simulink model "Microgrid_transition_model_092221"  (R2020a)
settings: Solver=VariableStepAuto  StartTime=0.0  StopTime=16  MaxStep=1e-4  RelTol=1e-3
PreLoadFcn:
  | %run('FC_microgrid_param.m')
  | %load('gen_grid_init.mat')
InitFcn:
  | %load myisoModel_init;
  | run('FC_microgrid_param.m')
  | tic
  | run('CARTinitFcn.m')
  | %caseNo = 2;
  | 
  | %if (caseNo == 1)
  | %set_param(['Isolated_grid_paper_model_022521/SignalGen'], 'ActiveScenario', 'PStep222kW');
  | %else
  | %set_param(['Isolated_grid_paper_model_022521/SignalGen'], 'ActiveScenario', 'QStep222kVAr');
  | 
  | %end;
StopFcn:
  | toc
undefined symbols (not defined in the file): breakpoints1, breakpoints2, cp_table_data, ctrl, D1, Delta, DiscIntNeverNeededParam, DT, FC_BESS, find_system, gcbh, libFC_BESS, LowerLimit, magnitude, oversize, pq_ts, sps_rtmsupport, timer, ts, Ts, Ts_APC, Ts_Control, Ts_Power, UpperLimit
libraries: powerlib x120, powerlib_meascontrol x85, simulink x63, powerlib_extras x40, simulink_extras x12, eePowerMeasurement x9, sps_avr x7, pi_ctrl x4, spsDieselMotorModel x3, SignalEditorBlockLib x2, libLgBattery x1, libFC_PV x1
(part 8 of 11)

== system Microgrid_transition_model_092221/../Control/Grid-side converter Control system/INT ==
  note: INTEGRATOR (Trapezoidal) with External limits & Reset & Hold
  Max : Inport
  Min : Inport  Port=2
  In : Inport  Port=3
  Ki : Inport  Port=4
  Hold : Inport  Port=5
  Reset : Inport  Port=6
  Reset Value : Inport  Port=7
  Gain : Gain  Gain=Ts* 0.5  SaturateOnIntegerOverflow=on  OutDataTypeStr=Inherit: Same as input  ParamDataTypeStr=Inherit: Same as input
  IC = 0 : UnitDelay  SampleTime=Ts  HasFrameUpgradeWarning=on
  IC = i_ic : UnitDelay  SampleTime=Ts  HasFrameUpgradeWarning=on
  Logical Operator4 : Logic  Operator=OR
  MinMax : MinMax  Inputs=2  InputSameDT=on  SaturateOnIntegerOverflow=on
  MinMax1 : MinMax  Function=max  Inputs=2  InputSameDT=on  SaturateOnIntegerOverflow=on
  Product : Product  SaturateOnIntegerOverflow=on  OutDataTypeStr=Inherit: Same as first input
  S6 : Subsystem  mask(Limiter with External Limits){}
      mask Display: disp('      Limiter\n')
  Sum : Sum  InputSameDT=on  SaturateOnIntegerOverflow=on  OutDataTypeStr=Inherit: Same as first input
  Sum1 : Sum  InputSameDT=on  SaturateOnIntegerOverflow=on  OutDataTypeStr=Inherit: Same as first input
  Switch2 : Switch  Threshold=0.5  SaturateOnIntegerOverflow=on  InputSameDT=on
  Switch3 : Switch  Threshold=0.5  SaturateOnIntegerOverflow=on  InputSameDT=on
  Switch7 : Switch  Threshold=0.5  SaturateOnIntegerOverflow=on  InputSameDT=on
  Out : Outport  InitialOutput=0  VectorParamsAs1DForOutWhenUnconnected=off
  wires:
  S6/1("  ") -> IC = i_ic/1, Out/1
  Gain/1 -> Product/1
  Sum1/1 -> Product/2
  Ki/1 -> Gain/1
  IC = 0/1 -> Sum1/2
  In/1 -> IC = 0/1, Sum1/1
  Product/1 -> Sum/1
  Sum/1 -> S6/2(In)
  Hold/1 -> Logical Operator4/1
  Reset/1 -> Switch7/2, Logical Operator4/2
  Logical Operator4/1 -> Switch2/2, Switch3/2
  Switch2/1 -> MinMax/1
  Max/1 -> Switch2/3, MinMax/2
  Reset Value/1 -> Switch7/1
  MinMax/1 -> S6/1(MAX)
  MinMax1/1 -> S6/3(MIN)
  Switch3/1 -> MinMax1/1
  Min/1 -> Switch3/3, MinMax1/2
  IC = i_ic/1 -> Switch7/3
  Switch7/1 -> Switch2/1, Sum/2, Switch3/1

== system Microgrid_transition_model_092221/../Control/Measurement and Transformation/Discrete 3-phase PLL-Driven Positive-Sequence Active & Reactive Power ==
  note: Discrete 3-phase PLL-driven Positive-Sequence Active & Reactive Power
  note: Pierre Giroux, Gilbert Sybille
      | Power System Simulation Laboratory
      | IREQ, Hydro-Quebc
  Freq : Inport  PortDimensions=1
  w : Inport  Port=2  PortDimensions=1
  Vabc : Inport  Port=3  PortDimensions=3
  Iabc : Inport  Port=4  PortDimensions=3
  Deg->Rad : Gain  Gain=pi/180  SaturateOnIntegerOverflow=on  OutDataTypeStr=Inherit: Same as input  ParamDataTypeStr=Inherit: Same as input
  Discrete 3-phase PLL-Driven Positive-Sequence Fundamental Value : Subsystem  mask(Discrete 3-phase PLL-Driven Positive-Sequence Fundamental Value){Finit=Finit, Fmin=Fmin, Par_Init=Par_Vinit, Ts=Ts}
      mask prompts: Finit "Initial frequency (Hz):"; Fmin "Minimum frequency (Hz):"; Par_Init "Initial input (positive component): [ Mag  Phase-relative-to-PLL(degrees) ]"; Ts "Sample time:"
      mask help:
      | For a supplied fundamental frequency (port Freq), this discrete block computes  the positive-sequence component (Magnitude and Phase)  of a set of three balanced or unbalanced signals (port abc) which may contain harmonics.
      |  Input port "Sin_Cos" (a two-dimension signal) provides the reference frame required for the computation..
      |  First and second outputs return respectively the magnitude and phase (in degrees relative to the PLL phase)) of the fundamental.
      | For the first cycle of simulation, the outputs are held constant to the values specified by the parameter "Initial input".
      | constant to the values specified by the parameter "Initial input". The value of the parameter "Minimum frequency" is used to determine the buffer size of the "Variable Transport Delay" block found inside this subsystem.
      mask init:
      | Real_Init=Par_Init(1)*cos(pi/180*Par_Init(2));
      | Imag_Init=Par_Init(1)*sin(pi/180*Par_Init(2));
      | power_initmask();
      settings: OpenFcn=power_openblockproxy();
  Discrete 3-phase PLL-Driven Positive-Sequence Fundamental Value2 : Subsystem  mask(Discrete 3-phase PLL-Driven Positive-Sequence Fundamental Value){Finit=Finit, Fmin=Fmin, Par_Init=Par_Iinit, Ts=Ts}
      mask prompts: Finit "Initial frequency (Hz):"; Fmin "Minimum frequency (Hz):"; Par_Init "Initial input (positive component): [ Mag  Phase-relative-to-PLL(degrees) ]"; Ts "Sample time:"
      mask help:
      | For a supplied fundamental frequency (port Freq), this discrete block computes  the positive-sequence component (Magnitude and Phase)  of a set of three balanced or unbalanced signals (port abc) which may contain harmonics.
      |  Input port "Sin_Cos" (a two-dimension signal) provides the reference frame required for the computation..
      |  First and second outputs return respectively the magnitude and phase (in degrees relative to the PLL phase)) of the fundamental.
      | For the first cycle of simulation, the outputs are held constant to the values specified by the parameter "Initial input".
      | constant to the values specified by the parameter "Initial input". The value of the parameter "Minimum frequency" is used to determine the buffer size of the "Variable Transport Delay" block found inside this subsystem.
      mask init:
      | Real_Init=Par_Init(1)*cos(pi/180*Par_Init(2));
      | Imag_Init=Par_Init(1)*sin(pi/180*Par_Init(2));
      | power_initmask();
      settings: OpenFcn=power_openblockproxy();
  Gain1 : Gain  Gain=3/2  SaturateOnIntegerOverflow=on  OutDataTypeStr=Inherit: Same as input  ParamDataTypeStr=Inherit: Same as input
  Mux2 : Mux  Inputs=2
  Mux3 : Mux  Inputs=2
  Product : Product  InputSameDT=on  SaturateOnIntegerOverflow=on  OutDataTypeStr=Inherit: Same as first input
  Product1 : Product  InputSameDT=on  SaturateOnIntegerOverflow=on  OutDataTypeStr=Inherit: Same as first input
  Product2 : Product  InputSameDT=on  SaturateOnIntegerOverflow=on  OutDataTypeStr=Inherit: Same as first input
  Sum : Sum  Inputs=+-  InputSameDT=on  SaturateOnIntegerOverflow=on  OutDataTypeStr=Inherit: Same as first input
  Trigonometric Function : Trigonometry
  Trigonometric Function1 : Trigonometry  Operator=cos
  Mag_V_I : Outport  VectorParamsAs1DForOutWhenUnconnected=off
  P_Q : Outport  Port=2  VectorParamsAs1DForOutWhenUnconnected=off
  wires:
  Vabc/1 -> Discrete 3-phase PLL-Driven Positive-Sequence Fundamental Value/3(abc)
  Freq/1 -> Discrete 3-phase PLL-Driven Positive-Sequence Fundamental Value/1(Freq), Discrete 3-phase PLL-Driven Positive-Sequence Fundamental Value2/1(Freq)
  w/1 -> Discrete 3-phase PLL-Driven Positive-Sequence Fundamental Value/2(w), Discrete 3-phase PLL-Driven Positive-Sequence Fundamental Value2/2(w)
  Discrete 3-phase PLL-Driven Positive-Sequence Fundamental Value/2(Phase) -> Sum/1
  Discrete 3-phase PLL-Driven Positive-Sequence Fundamental Value/1(Mag) -> Mux3/1, Product2/1
  Discrete 3-phase PLL-Driven Positive-Sequence Fundamental Value2/2(Phase) -> Sum/2
  Sum/1 -> Deg->Rad/1
  Deg->Rad/1 -> Trigonometric Function1/1, Trigonometric Function/1
  Trigonometric Function1/1 -> Product/2
  Trigonometric Function/1 -> Product1/1
  Mux2/1 -> Gain1/1
  Product/1 -> Mux2/1
  Product1/1 -> Mux2/2
  Mux3/1 -> Mag_V_I/1
  Gain1/1 -> P_Q/1
  Product2/1 -> Product/1, Product1/2
  Discrete 3-phase PLL-Driven Positive-Sequence Fundamental Value2/1(Mag) -> Mux3/2, Product2/2
  Iabc/1 -> Discrete 3-phase PLL-Driven Positive-Sequence Fundamental Value2/3(abc)

== system Microgrid_transition_model_092221/../Control/Measurement and Transformation/Filter ==
  Vabc_grid : Inport
  Iabc_grid_conv : Inport  Port=2
  Vabc_LL_s : Inport  Port=3
  Iabc_stator : Inport  Port=4
  IL : Inport  Port=5
  Vdc : Inport  Port=6
  Qref : Inport  Port=7
  wr : Inport  Port=8
  angle_rotor : Inport  Port=9
  Second-Order Filter{,1..6} (7 alike) : powerlib_meascontrol/Filters/Second-Order Filter  FilterType=Lowpass  Fo=Freq  Zeta=Zeta  Ts=Ts  Initialize=off  Vac_Init="[0,  0,  60]"  Vdc_Init=0  PlotResponse=off  FreqRange=[0, 500, 1]
      settings: SourceProductBaseCode=MT,PS
  Second-Order Filter7 : powerlib_meascontrol/Filters/Second-Order Filter  FilterType=Lowpass  Fo=Freq  Zeta=Zeta  Ts=Ts  Initialize=on  Vac_Init=[0.8 -25 60]*0  Vdc_Init=Vdc_nom  PlotResponse=off  FreqRange=[0, 500, 1]
      settings: SourceProductBaseCode=MT,PS
  Second-Order Filter8 : powerlib_meascontrol/Filters/Second-Order Filter  FilterType=Lowpass  Fo=Freq  Zeta=Zeta  Ts=Ts  Initialize=on  Vac_Init=[0.8 -25 60]*0  Vdc_Init=1+init(1)/100  PlotResponse=off  FreqRange=[0, 500, 1]
      settings: SourceProductBaseCode=MT,PS
  "Vabc_grid " : Outport  VectorParamsAs1DForOutWhenUnconnected=off
  "Iabc_grid_conv " : Outport  Port=2  VectorParamsAs1DForOutWhenUnconnected=off
  "Vabc_LL_s " : Outport  Port=3  VectorParamsAs1DForOutWhenUnconnected=off
  "Iabc_stator " : Outport  Port=4  VectorParamsAs1DForOutWhenUnconnected=off
  "IL " : Outport  Port=5  VectorParamsAs1DForOutWhenUnconnected=off
  "Vdc " : Outport  Port=6  VectorParamsAs1DForOutWhenUnconnected=off
  "Qref " : Outport  Port=7  VectorParamsAs1DForOutWhenUnconnected=off
  "wr " : Outport  Port=8  VectorParamsAs1DForOutWhenUnconnected=off
  "angle_rotor " : Outport  Port=9  VectorParamsAs1DForOutWhenUnconnected=off
  wires:
  Iabc_stator/1 -> Second-Order Filter3/1
  Second-Order Filter2/1 -> "Vabc_LL_s "/1
  Vabc_LL_s/1 -> Second-Order Filter2/1
  Iabc_grid_conv/1 -> Second-Order Filter1/1
  Vabc_grid/1 -> Second-Order Filter/1
  Second-Order Filter4/1 -> "IL "/1
  IL/1 -> Second-Order Filter4/1
  Second-Order Filter5/1 -> "Qref "/1
  Qref/1 -> Second-Order Filter5/1
  Second-Order Filter8/1 -> "wr "/1
  wr/1 -> Second-Order Filter8/1
  Second-Order Filter3/1 -> "Iabc_stator "/1
  Second-Order Filter7/1 -> "Vdc "/1
  Vdc/1 -> Second-Order Filter7/1
  Second-Order Filter1/1 -> "Iabc_grid_conv "/1
  Second-Order Filter/1 -> "Vabc_grid "/1
  Second-Order Filter6/1 -> "angle_rotor "/1
  angle_rotor/1 -> Second-Order Filter6/1

== system Microgrid_transition_model_092221/../Control/Measurement and Transformation/Stator flux estimator ==
  note: Quasi steady state flux at generator stator
  Vdqs : Inport
  Idqs : Inport  Port=2
  wr : Inport  Port=3
  Divide2 : Product  Inputs=**
  Divide4 : Product  Inputs=*/
  Divide7 : Product  Inputs=**
  Divide8 : Product  Inputs=*/
  First-Order Filter : powerlib_meascontrol/Filters/First-Order Filter  FilterType=Lowpass  Tc=Flux_meas_time_constant  Ts=Ts  Initialize=on  Vac_Init=[0, 0, 0]  Vdc_Init=1  PlotResponse=off  FreqRange="[0,  200,  1]"
      settings: SourceProductBaseCode=MT,PS
  Gain : Gain  Gain=-1
  Magnitude of flux : Fcn  Expr=sqrt(u(1)^2+u(2)^2)
  Mux1 : Mux  Inputs=2
  Rs2 : Constant  Value=Resistance
  Rs4 : Constant  Value=Resistance
  Selector1 : Selector  InputPortWidth=2  IndexOptions=Index vector (dialog)  Indices=2  OutputSizes=1
  Selector3 : Selector  InputPortWidth=2  IndexOptions=Index vector (dialog)  Indices=2  OutputSizes=1
  Selector7 : Selector  InputPortWidth=2  IndexOptions=Index vector (dialog)  Indices=1  OutputSizes=1
  Selector8 : Selector  InputPortWidth=2  IndexOptions=Index vector (dialog)  Indices=1  OutputSizes=1
  Sum2 : Sum  Inputs=|+-
  Sum4 : Sum  Inputs=|+-
  avoid division by 0 : Saturate  UpperLimit=inf  LowerLimit=1e-6
  Flux : Outport  VectorParamsAs1DForOutWhenUnconnected=off
  wires:
  wr/1 -> avoid division by 0/1
  Sum2/1 -> Divide4/1
  Divide4/1 -> Mux1/1  "phi_d"
  Divide2/1 -> Sum2/2  "Rs*Iq"
  Selector1/1 -> Sum2/1  "Vq"
  Rs2/1 -> Divide2/2
  Selector3/1 -> Divide2/1  "Iq"
  Vdqs/1 -> Selector1/1, Selector7/1
  Idqs/1 -> Selector3/1, Selector8/1
  Divide7/1 -> Sum4/2  "Rs*Id"
  Selector7/1 -> Sum4/1  "Vd"
  Rs4/1 -> Divide7/2
  Selector8/1 -> Divide7/1  "Id"
  Sum4/1 -> Divide8/1
  Gain/1 -> Divide8/2
  Divide8/1 -> Mux1/2  "phi_q"
  Mux1/1 -> Magnitude of flux/1
  Magnitude of flux/1 -> First-Order Filter/1
  avoid division by 0/1 -> Divide4/2, Gain/1
  First-Order Filter/1 -> Flux/1

== system Microgrid_transition_model_092221/../Control/Measurement and Transformation/abc2qd ==
  note: This subsystem converts Vab and Vbc to Vd,Vq. The sine and cosine com-
      | puted here are sent to the inverse transformation subsystem qd/abc.
  Vabc_LL : Inport
  sin_cos : Inport  Port=2
  Fcn2 : Fcn  Expr=(u[4]*(2*u[1]+u[2]) + (sqrt(3)*u[2]*u[3])) * 1/3
  Fcn3 : Fcn  Expr=(u[3]*(2*u[1]+u[2]) + (-sqrt(3)*u[2]*u[4])) * 1/3
  Mux : Mux  Inputs=2
  Mux1 : Mux  Inputs=[ 2 2 ]
  Selector : Selector  InputPortWidth=3  IndexOptions=Index vector (dialog)  Indices=[1 2]  OutputSizes=1
  Vdq : Outport  InitialOutput=0  VectorParamsAs1DForOutWhenUnconnected=off
  wires:
  Selector/1 -> Mux1/1
  Mux/1 -> Vdq/1
  sin_cos/1 -> Mux1/2
  Vabc_LL/1 -> Selector/1
  Mux1/1 -> Fcn2/1, Fcn3/1
  Fcn2/1 -> Mux/2
  Fcn3/1 -> Mux/1

== system Microgrid_transition_model_092221/../Control/Speed & Pitch Control/Discrete PI Controller ==
  note: Pierre Giroux, Gilbert Sybille
      | Power System Simulation Laboratory
      | IREQ, Hydro-Quebc
  note: Discrete PID Controller
  Error : Inport  SampleTime=Ts
  Discrete-Time Integrator : DiscreteIntegrator  InitialCondition=Init  SampleTime=Ts  LimitOutput=on  UpperSaturationLimit=UpperLimit  LowerSaturationLimit=LowerLimit  ICPrevOutput=DiscIntNeverNeededParam  ICPrevScaledInput=DiscIntNeverNeededParam
  Kp4 : Gain  Gain=Kp  SaturateOnIntegerOverflow=on  SampleTime=Ts  OutDataTypeStr=Inherit: Same as input  ParamDataTypeStr=Inherit: Same as input
  Kp5 : Gain  Gain=Ki  SaturateOnIntegerOverflow=on  SampleTime=Ts  OutDataTypeStr=Inherit: Same as input  ParamDataTypeStr=Inherit: Same as input
  Saturation2 : Saturate  UpperLimit=UpperLimit  LowerLimit=LowerLimit  SampleTime=Ts
  Sum6 : Sum  InputSameDT=on  SaturateOnIntegerOverflow=on  SampleTime=Ts  OutDataTypeStr=Inherit: Same as first input
  Zero-Order Hold : ZeroOrderHold  SampleTime=Ts
  Out : Outport  SampleTime=Ts  InitialOutput=0  VectorParamsAs1DForOutWhenUnconnected=off
  wires:
  Error/1 -> Kp4/1, Kp5/1
  Sum6/1 -> Saturation2/1
  Kp5/1 -> Discrete-Time Integrator/1
  Kp4/1 -> Zero-Order Hold/1
  Discrete-Time Integrator/1 -> Sum6/2
  Saturation2/1 -> Out/1
  Zero-Order Hold/1 -> Sum6/1

== system Microgrid_transition_model_092221/../Control/Speed & Pitch Control/Discrete PI Controller1 ==
  note: Pierre Giroux, Gilbert Sybille
      | Power System Simulation Laboratory
      | IREQ, Hydro-Quebc
  note: Discrete PID Controller
  Error : Inport  SampleTime=Ts
  Discrete-Time Integrator : DiscreteIntegrator  InitialCondition=Init  SampleTime=Ts  LimitOutput=on  UpperSaturationLimit=UpperLimit  LowerSaturationLimit=LowerLimit  ICPrevOutput=DiscIntNeverNeededParam  ICPrevScaledInput=DiscIntNeverNeededParam
  Kp4 : Gain  Gain=Kp  SaturateOnIntegerOverflow=on  SampleTime=Ts  OutDataTypeStr=Inherit: Same as input  ParamDataTypeStr=Inherit: Same as input
  Kp5 : Gain  Gain=Ki  SaturateOnIntegerOverflow=on  SampleTime=Ts  OutDataTypeStr=Inherit: Same as input  ParamDataTypeStr=Inherit: Same as input
  Saturation2 : Saturate  UpperLimit=UpperLimit  LowerLimit=LowerLimit  SampleTime=Ts
  Sum6 : Sum  InputSameDT=on  SaturateOnIntegerOverflow=on  SampleTime=Ts  OutDataTypeStr=Inherit: Same as first input
  Zero-Order Hold : ZeroOrderHold  SampleTime=Ts
  Out : Outport  SampleTime=Ts  InitialOutput=0  VectorParamsAs1DForOutWhenUnconnected=off
  wires:
  Error/1 -> Kp4/1, Kp5/1
  Sum6/1 -> Saturation2/1
  Kp5/1 -> Discrete-Time Integrator/1
  Kp4/1 -> Zero-Order Hold/1
  Discrete-Time Integrator/1 -> Sum6/2
  Saturation2/1 -> Out/1
  Zero-Order Hold/1 -> Sum6/1

== system Microgrid_transition_model_092221/../Control/Speed & Pitch Control/Discrete PI Controller2 ==
  note: Pierre Giroux, Gilbert Sybille
      | Power System Simulation Laboratory
      | IREQ, Hydro-Quebc
  note: Discrete PID Controller
  Error : Inport  SampleTime=Ts
  Discrete-Time Integrator : DiscreteIntegrator  InitialCondition=Init  SampleTime=Ts  LimitOutput=on  UpperSaturationLimit=UpperLimit  LowerSaturationLimit=LowerLimit  ICPrevOutput=DiscIntNeverNeededParam  ICPrevScaledInput=DiscIntNeverNeededParam
  Kp4 : Gain  Gain=Kp  SaturateOnIntegerOverflow=on  SampleTime=Ts  OutDataTypeStr=Inherit: Same as input  ParamDataTypeStr=Inherit: Same as input
  Kp5 : Gain  Gain=Ki  SaturateOnIntegerOverflow=on  SampleTime=Ts  OutDataTypeStr=Inherit: Same as input  ParamDataTypeStr=Inherit: Same as input
  Saturation2 : Saturate  UpperLimit=UpperLimit  LowerLimit=LowerLimit  SampleTime=Ts
  Sum6 : Sum  InputSameDT=on  SaturateOnIntegerOverflow=on  SampleTime=Ts  OutDataTypeStr=Inherit: Same as first input
  Zero-Order Hold : ZeroOrderHold  SampleTime=Ts
  Out : Outport  SampleTime=Ts  InitialOutput=0  VectorParamsAs1DForOutWhenUnconnected=off
  wires:
  Error/1 -> Kp4/1, Kp5/1
  Sum6/1 -> Saturation2/1
  Kp5/1 -> Discrete-Time Integrator/1
  Kp4/1 -> Zero-Order Hold/1
  Discrete-Time Integrator/1 -> Sum6/2
  Saturation2/1 -> Out/1
  Zero-Order Hold/1 -> Sum6/1

== system Microgrid_transition_model_092221/FC_BESS/SMAInverter/85_SMAControl/InvControl ==
  Uabc : Inport  PortDimensions=3
  Uabc_inv : Inport  Port=2  PortDimensions=3
  Iabc : Inport  Port=3  PortDimensions=3
  cb_stat : Inport  Port=4  OutDataTypeStr=double
  pref : Inport  Port=5
  qref : Inport  Port=6
  fref : Inport  Port=7
  vref : Inport  Port=8
  GF_mode_en : Inport  Port=9
  40_V_Control : Subsystem
  50_I_Control : Subsystem
  Bus Creator : BusCreator  Inputs=11
  Bus Creator1 : BusCreator  Inputs=3
  Bus Selector : BusSelector  OutputSignals=Uabc_ref
  CB_Meas2 : Subsystem
  CB_pu : Subsystem
  CS_controller : Subsystem
  Constant : Constant  Value=0.016666/2.3
  Constant1 : Constant  Value=0.05/2.3
  Constant3 : Constant  Value=0  OutDataTypeStr=boolean
  Constant4 : Constant  OutDataTypeStr=boolean
  Droop : Subsystem
  Goto Tag Visibility1 : GotoTagVisibility  GotoTag=inputs
  Goto Tag Visibility10 : GotoTagVisibility  GotoTag=I_Ctrl
  Goto Tag Visibility2 : GotoTagVisibility  GotoTag=cb_meas
  Goto Tag Visibility4 : GotoTagVisibility  GotoTag=droop
  Goto Tag Visibility5 : GotoTagVisibility  GotoTag=inverter
  Goto Tag Visibility6 : GotoTagVisibility  GotoTag=cb_pu
  Goto Tag Visibility7 : GotoTagVisibility  GotoTag=pll
  Goto Tag Visibility8 : GotoTagVisibility  GotoTag=ref_lim
  Goto Tag Visibility9 : GotoTagVisibility  GotoTag=V_Ctrl
  PLL : Subsystem
  Ref_Limiting : Subsystem
  Uabc_ref : Outport  VectorParamsAs1DForOutWhenUnconnected=off
  tag scope: inputs=scoped
  wires:
  Constant1/1 -> Bus Creator/10  "VQ_droop"
  cb_stat/1 -> Bus Creator/6  "cb_status"
  Uabc/1 -> Bus Creator/1  "Uabc"
  Bus Creator/1 -> [inputs]
  vref/1 -> Bus Creator/8  "vref"
  [inverter] -> Bus Selector/1
  Iabc/1 -> Bus Creator/3  "Iabc"
  fref/1 -> Bus Creator/7  "fref"
  Bus Selector/1 -> Uabc_ref/1  "<Uabc_ref>"
  Constant3/1 -> Bus Creator1/3  "Reset"
  Constant4/1 -> Bus Creator1/2  "Enable"
  GF_mode_en/1 -> Bus Creator1/1  "GF_mode"
  Bus Creator1/1 -> Bus Creator/11  "Control_Word"
  Constant/1 -> Bus Creator/9  "FP_droop"
  qref/1 -> Bus Creator/5  "qref"
  pref/1 -> Bus Creator/4  "pref"
  Uabc_inv/1 -> Bus Creator/2  "Uabc_inv"

== system Microgrid_transition_model_092221/Grid Feeder Protective Relay/R25 - Sync Check v0.1/Phase_Comparator/WrapPi ==
  In1 : Inport
  Compare To Constant1 : simulink/Logic and Bit Operations/Compare To Constant  relop=<=  const=-pi  OutDataTypeStr=boolean
  Compare To Constant2 : simulink/Logic and Bit Operations/Compare To Constant  relop=>=  const=pi  OutDataTypeStr=boolean
  Gain1 : Gain  Gain=2*pi
  Gain2 : Gain  Gain=2*pi
  Sum : Sum  Inputs=++-
  Out1 : Outport
  wires:
  Compare To Constant2/1 -> Gain2/1
  Compare To Constant1/1 -> Gain1/1
  In1/1 -> Sum/2, Compare To Constant1/1, Compare To Constant2/1
  Gain2/1 -> Sum/3
  Gain1/1 -> Sum/1
  Sum/1 -> Out1/1

== system Microgrid_transition_model_092221/Grid Feeder Protective Relay1/R25 - Sync Check v0.1/Phase_Comparator/WrapPi ==
  In1 : Inport
  Compare To Constant1 : simulink/Logic and Bit Operations/Compare To Constant  relop=<=  const=-pi  OutDataTypeStr=boolean
  Compare To Constant2 : simulink/Logic and Bit Operations/Compare To Constant  relop=>=  const=pi  OutDataTypeStr=boolean
  Gain1 : Gain  Gain=2*pi
  Gain2 : Gain  Gain=2*pi
  Sum : Sum  Inputs=++-
  Out1 : Outport
  wires:
  Sum/1 -> Out1/1
  Gain1/1 -> Sum/1
  Gain2/1 -> Sum/3
  In1/1 -> Compare To Constant2/1, Compare To Constant1/1, Sum/2
  Compare To Constant1/1 -> Gain1/1
  Compare To Constant2/1 -> Gain2/1

== system Microgrid_transition_model_092221/Wind Turbine Type 4/APC (atomic)1/Inertial Response (to df)/FBIC ==
  wg (pu) : Inport
  Freq (Hz)1 : Inport  Port=2
  Act1 : Inport  Port=3
  Discrete Transfer Fcn : DiscreteTransferFcn  Numerator=[0.99985 -0.99985]  Denominator=[1 -0.99985]
  Display3 : Display
  Display4 : Display
  FBIC performance1 : Scope  NumInputPorts=2
  Logical Operator1 : Logic  Operator=NOT  AllPortsSameDT=off  OutDataTypeStr=boolean
  Low-Pass Filter 1 : eeGeneralControl/Low-Pass Filter (Discrete or Continuous)  K=1  T=1  B=inf  A=-inf  init_option=Inherited from block input  x0=0  Ts=-1
  Nominal F1 : Constant
  S&H1 : Subsystem  mask{ic=0}
      mask prompts: ic "Initial condition"
  Saturation1 : Saturate  UpperLimit=0.3  LowerLimit=0
  Sum1 : Sum  Inputs=+-|
  adaptive FBIC1 : MATLAB Function  TreatAsAtomicUnit=on
  inertial1 : simulink/Discrete/Discrete Derivative  gainval=1.0  ICPrevScaledInput=1  OutMin=[]  OutMax=[]  OutDataType=fixdt(1, 16)  OutScaling=2^-10  DoSatur=off
  to pu 1 : Gain  Gain=1/60
  Delta_P FBIC1 : Outport
  wires:
  inertial1/1 -> adaptive FBIC1/1(F_de), Display3/1
  adaptive FBIC1/3(P_dr) -> FBIC performance1/2
  adaptive FBIC1/2(P_de) -> FBIC performance1/1
  Freq (Hz)1/1 -> to pu 1/1
  S&H1/1(Out) -> adaptive FBIC1/3(Wi)
  Act1/1 -> adaptive FBIC1/4(Act), Logical Operator1/1
  wg (pu)/1 -> S&H1/1(In)
  adaptive FBIC1/1(Delta_P) -> Saturation1/1
  Logical Operator1/1 -> S&H1/2(S)
  Low-Pass Filter 1/1 -> inertial1/1, Display4/1
  Nominal F1/1 -> Sum1/2
  Saturation1/1 -> Delta_P FBIC1/1
  Sum1/1 -> Discrete Transfer Fcn/1
  to pu 1/1 -> Sum1/1, Low-Pass Filter 1/1
  Discrete Transfer Fcn/1 -> adaptive FBIC1/2(F_dr)

== system Microgrid_transition_model_092221/Wind Turbine Type 4/APC (atomic)1/Inertial Response (to df)/Lock2 ==
  I : Inport
  R : Inport  Port=2
  Constant7 : Constant  Value=0
  Display1 : Display
  Display16 : Display
  Freq Act : Switch  Threshold=0.5
  Logical Operator1 : Logic  Operator=NOT  AllPortsSameDT=off  OutDataTypeStr=boolean
  Logical Operator3 : Logic  Operator=NOT  AllPortsSameDT=off  OutDataTypeStr=boolean
  S&H : Subsystem  mask{ic=0}
      mask prompts: ic "Initial condition"
  Unit Delay : UnitDelay  SampleTime=-1  HasFrameUpgradeWarning=on
  O : Outport
  wires:
  Logical Operator1/1 -> Freq Act/2, Display16/1
  R/1 -> Logical Operator1/1
  Constant7/1 -> Freq Act/3
  Freq Act/1 -> Logical Operator3/1
  S&H/1(Out) -> O/1, Display1/1, Freq Act/1
  I/1 -> S&H/1(In)
  Logical Operator3/1 -> Unit Delay/1
  Unit Delay/1 -> S&H/2(S)

== system Microgrid_transition_model_092221/Wind Turbine Type 4/APC (atomic)1/Inertial Response (to df)/TLIC ==
  Act : Inport
  Delay1 : Delay  DelayLength=1  InitialCondition=0
  Delay2 : Delay  DelayLength=1  InitialCondition=0
  Delay3 : Delay  DelayLength=1  InitialCondition=0
  Display1 : Display
  Display2 : Display
  Scope : Scope  NumInputPorts=4
  adaptive TLIC : MATLAB Function  TreatAsAtomicUnit=on
  Delta_P TLIC : Outport
  wires:
  Delay3/1 -> Scope/2, adaptive TLIC/1("recharge ")  "recharge"
  Delay2/1 -> adaptive TLIC/2("trecharge "), Scope/3  "trecharge"
  Delay1/1 -> adaptive TLIC/3("tIR "), Scope/4  "tIR"
  adaptive TLIC/4(tIR) -> Delay1/1
  adaptive TLIC/3(trecharge) -> Delay2/1
  adaptive TLIC/2(recharge) -> Delay3/1
  Act/1 -> adaptive TLIC/4(Act), Display2/1
  adaptive TLIC/1(Delta_P) -> Delta_P TLIC/1, Display1/1, Scope/1  "dP"

== system Microgrid_transition_model_092221/Wind Turbine Type 4/Control/Excitation Control system/Discrete PI Controller ==
  note: Discrete PID Controller
  note: Pierre Giroux, Gilbert Sybille
      | Power System Simulation Laboratory
      | IREQ, Hydro-Quebc
  Error : Inport  SampleTime=Ts
  Discrete-Time Integrator : DiscreteIntegrator  InitialCondition=Init  SampleTime=Ts  LimitOutput=on  UpperSaturationLimit=UpperLimit  LowerSaturationLimit=LowerLimit  ICPrevOutput=DiscIntNeverNeededParam  ICPrevScaledInput=DiscIntNeverNeededParam
  Kp4 : Gain  Gain=Kp  SaturateOnIntegerOverflow=on  SampleTime=Ts  OutDataTypeStr=Inherit: Same as input  ParamDataTypeStr=Inherit: Same as input
  Kp5 : Gain  Gain=Ki  SaturateOnIntegerOverflow=on  SampleTime=Ts  OutDataTypeStr=Inherit: Same as input  ParamDataTypeStr=Inherit: Same as input
  Saturation2 : Saturate  UpperLimit=UpperLimit  LowerLimit=LowerLimit  SampleTime=Ts
  Sum6 : Sum  InputSameDT=on  SaturateOnIntegerOverflow=on  SampleTime=Ts  OutDataTypeStr=Inherit: Same as first input
  Zero-Order Hold : ZeroOrderHold  SampleTime=Ts
  Out : Outport  SampleTime=Ts  InitialOutput=0  VectorParamsAs1DForOutWhenUnconnected=off
  wires:
  Zero-Order Hold/1 -> Sum6/1
  Saturation2/1 -> Out/1
  Discrete-Time Integrator/1 -> Sum6/2
  Kp4/1 -> Zero-Order Hold/1
  Kp5/1 -> Discrete-Time Integrator/1
  Sum6/1 -> Saturation2/1
  Error/1 -> Kp5/1, Kp4/1

== system Microgrid_transition_model_092221/Wind Turbine Type 4/Control/Grid-Side Inverter Control/Counter AST ==
  Trigger : TriggerPort  VariantControl=Variant  PortDimensions=1
  Constant : Constant
  Memory : Memory  InheritSampleTime=on
  Sum : Sum  Inputs=|++
  Count : Outport
  wires:
  Constant/1 -> Sum/2
  Sum/1 -> Memory/1, Count/1
  Memory/1 -> Sum/1

== system Microgrid_transition_model_092221/Wind Turbine Type 4/Control/Grid-Side Inverter Control/Discrete PI Controller1 ==
  note: Discrete PID Controller
  note: Pierre Giroux, Gilbert Sybille
      | Power System Simulation Laboratory
      | IREQ, Hydro-Quebc
  Error : Inport  SampleTime=Ts
  Discrete-Time Integrator : DiscreteIntegrator  InitialCondition=Init  SampleTime=Ts  LimitOutput=on  UpperSaturationLimit=UpperLimit  LowerSaturationLimit=LowerLimit  ICPrevOutput=DiscIntNeverNeededParam  ICPrevScaledInput=DiscIntNeverNeededParam
  Kp4 : Gain  Gain=Kp  SaturateOnIntegerOverflow=on  SampleTime=Ts  OutDataTypeStr=Inherit: Same as input  ParamDataTypeStr=Inherit: Same as input
  Kp5 : Gain  Gain=Ki  SaturateOnIntegerOverflow=on  SampleTime=Ts  OutDataTypeStr=Inherit: Same as input  ParamDataTypeStr=Inherit: Same as input
  Saturation2 : Saturate  UpperLimit=UpperLimit  LowerLimit=LowerLimit  SampleTime=Ts
  Sum6 : Sum  InputSameDT=on  SaturateOnIntegerOverflow=on  SampleTime=Ts  OutDataTypeStr=Inherit: Same as first input
  Zero-Order Hold : ZeroOrderHold  SampleTime=Ts
  Out : Outport  SampleTime=Ts  InitialOutput=0  VectorParamsAs1DForOutWhenUnconnected=off
  wires:
  Zero-Order Hold/1 -> Sum6/1
  Saturation2/1 -> Out/1
  Discrete-Time Integrator/1 -> Sum6/2
  Kp4/1 -> Zero-Order Hold/1
  Kp5/1 -> Discrete-Time Integrator/1
  Sum6/1 -> Saturation2/1
  Error/1 -> Kp5/1, Kp4/1

== system Microgrid_transition_model_092221/Wind Turbine Type 4/Control/Grid-Side Inverter Control/FRT_ramp_p ==
  note: Aramis Schwanka Trevisan adapted from:
      | Beat Ronner
      | ABB Industrie AG
      | Turgi, Switzerland
  UpperLimit : Inport
  u : Inport  Port=2
  LowerLimit : Inport  Port=3
  Saturation : simulink/Discontinuities/Saturation Dynamic  OutMin=[]  OutMax=[]  OutDataTypeStr=Inherit: Same as second input  OutDataType=fixdt(1, 16)  OutScaling=2^-10  DoSatur=off
  Sum : Sum  Inputs=|++  InputSameDT=on  SaturateOnIntegerOverflow=on  OutDataTypeStr=Inherit: Same as first input
  Sum7 : Sum  Inputs=|+-  InputSameDT=on  SaturateOnIntegerOverflow=on  OutDataTypeStr=Inherit: Same as first input
  Unit Delay : UnitDelay  InitialCondition=1  SampleTime=Ts  HasFrameUpgradeWarning=on
  l Ts : Gain  Gain=Ts
  u Ts : Gain  Gain=Ts
  y : Outport
  wires:
  Sum7/1 -> Saturation/2
  Saturation/1 -> Sum/1
  UpperLimit/1 -> u Ts/1
  LowerLimit/1 -> l Ts/1
  Sum/1 -> Unit Delay/1, y/1  "y"
  Unit Delay/1 -> Sum/2, Sum7/2  "y-1"
  u/1 -> Sum7/1
  u Ts/1 -> Saturation/1
  l Ts/1 -> Saturation/3

== system Microgrid_transition_model_092221/Wind Turbine Type 4/Control/Grid-Side Inverter Control/FRT_ramp_q ==
  note: Aramis Schwanka Trevisan adapted from:
      | Beat Ronner
      | ABB Industrie AG
      | Turgi, Switzerland
  UpperLimit : Inport
  u : Inport  Port=2
  LowerLimit : Inport  Port=3
  Saturation : simulink/Discontinuities/Saturation Dynamic  OutMin=[]  OutMax=[]  OutDataTypeStr=Inherit: Same as second input  OutDataType=fixdt(1, 16)  OutScaling=2^-10  DoSatur=off
  Sum : Sum  Inputs=|++  InputSameDT=on  SaturateOnIntegerOverflow=on  OutDataTypeStr=Inherit: Same as first input
  Sum7 : Sum  Inputs=|+-  InputSameDT=on  SaturateOnIntegerOverflow=on  OutDataTypeStr=Inherit: Same as first input
  Unit Delay : UnitDelay  InitialCondition=1  SampleTime=Ts  HasFrameUpgradeWarning=on
  l Ts : Gain  Gain=Ts
  u Ts : Gain  Gain=Ts
  y : Outport
  wires:
  l Ts/1 -> Saturation/3
  u Ts/1 -> Saturation/1
  u/1 -> Sum7/1
  Unit Delay/1 -> Sum7/2, Sum/2  "y-1"
  Sum/1 -> y/1, Unit Delay/1  "y"
  LowerLimit/1 -> l Ts/1
  UpperLimit/1 -> u Ts/1
  Saturation/1 -> Sum/1
  Sum7/1 -> Saturation/2

== system Microgrid_transition_model_092221/Wind Turbine Type 4/Control/Grid-Side Inverter Control/PI with anti-windup and dynamic limits - Id ==
  note: Aramis Schwanka Trevisan - 16.08.2016
      | PI-controller with anti-windup and dynamic limits
      | Update 17.12.2016: External reset
      | Update 21.02.2017: External reset + limitation
  UpperLimit : Inport
  Input : Inport  Port=2
  LowerLimit : Inport  Port=3
  Reset : Inport  Port=4
  x_reset : Inport  Port=5
  Add1 : Sum
  Add2 : Sum
  Add3 : Sum  Inputs=+++
  Compare To Zero : simulink/Logic and Bit Operations/Compare To Zero  relop=>  OutDataTypeStr=uint8  ZeroCross=off
  Compare To Zero1 : simulink/Logic and Bit Operations/Compare To Zero  relop=<  OutDataTypeStr=uint8  ZeroCross=off
  Constant : Constant  Value=0
  Discrete Integrator : DiscreteIntegrator  IntegratorMethod=Integration: Trapezoidal  gainval=1  ExternalReset=sampled level  InitialConditionSource=external  InitialCondition=Init  SampleTime=Ts  UpperSaturationLimit=UpperLimit  LowerSaturationLimit=LowerLimit  ShowStatePort=on  ICPrevOutput=DiscIntNeverNeededParam  ICPrevScaledInput=DiscIntNeverNeededParam
  IC : InitialCondition  Value=Init
  Kp1 : Gain  Gain=Kp  SaturateOnIntegerOverflow=on  SampleTime=Ts  OutDataTypeStr=Inherit: Same as input  ParamDataTypeStr=Inherit: Same as input
  Kp5 : Gain  Gain=Ki  SaturateOnIntegerOverflow=on  SampleTime=Ts  OutDataTypeStr=Inherit: Same as input  ParamDataTypeStr=Inherit: Same as input
  Logical Operator : Logic  AllPortsSameDT=off  OutDataTypeStr=boolean
  Logical Operator1 : Logic  AllPortsSameDT=off  OutDataTypeStr=boolean
  Logical Operator2 : Logic  Operator=OR  AllPortsSameDT=off  OutDataTypeStr=boolean
  Logical Operator3 : Logic  Operator=OR  Inputs=3  AllPortsSameDT=off  OutDataTypeStr=boolean
  Logical Operator4 : Logic  Operator=NOT  Inputs=3  AllPortsSameDT=off  OutDataTypeStr=boolean
  Product : Product  Inputs=3
  Product1 : Product  Inputs=3
  Product2 : Product
  Relational Operator : RelationalOperator  OutDataTypeStr=boolean  RndMeth=Nearest
  Relational Operator1 : RelationalOperator  Operator=<=  OutDataTypeStr=boolean  RndMeth=Nearest
  Relational Operator2 : RelationalOperator  OutDataTypeStr=boolean  RndMeth=Nearest
  Relational Operator3 : RelationalOperator  Operator=<=  OutDataTypeStr=boolean  RndMeth=Nearest
  Saturation Dynamic : simulink/Discontinuities/Saturation Dynamic  OutMin=[]  OutMax=[]  OutDataTypeStr=Inherit: Same as second input  OutDataType=fixdt(1, 16)  OutScaling=2^-10  DoSatur=off
  Scope3 : Scope
  Switch : Switch  Criteria=u2 > Threshold
  Zero-Order Hold : ZeroOrderHold  SampleTime=Ts
  Output : Outport
  wires:
  Reset/1 -> Scope3/1, Product2/2, Logical Operator3/3, Logical Operator4/1
  IC/1 -> Discrete Integrator/3
  Switch/1 -> Discrete Integrator/1
  Compare To Zero1/1 -> Logical Operator1/2  "Error_is_negative"
  Logical Operator/1 -> Logical Operator2/1
  Relational Operator/1 -> Logical Operator/1  "UpperLimit_is_Reached"
  Relational Operator1/1 -> Logical Operator1/1  "LowerLimit_Is_Reached"
  Saturation Dynamic/1 -> Output/1
  Logical Operator2/1 -> Switch/2
  Constant/1 -> Switch/1
  Kp5/1 -> Switch/3
  Add2/1 -> Saturation Dynamic/2
  Kp1/1 -> Zero-Order Hold/1
  Add1/1 -> Relational Operator/1, Relational Operator1/1
  Input/1 -> Kp5/1, Compare To Zero1/1, Compare To Zero/1, Kp1/1
  Compare To Zero/1 -> Logical Operator/2  "Error_is_positive"
  Logical Operator1/1 -> Logical Operator2/2
  Relational Operator2/1 -> Logical Operator3/1, Product/2
  Relational Operator3/1 -> Product1/2, Logical Operator3/2
  Logical Operator3/1 -> Discrete Integrator/2
  Add3/1 -> IC/1
  Product1/1 -> Add3/2
  UpperLimit/1 -> Saturation Dynamic/1, Relational Operator/2, Product/1, Relational Operator2/2
  Discrete Integrator/State -> Add1/1, Relational Operator3/1, Relational Operator2/1
  Discrete Integrator/1 -> Add2/2
  Logical Operator4/1 -> Product/3, Product1/1
  LowerLimit/1 -> Saturation Dynamic/3, Relational Operator1/2, Relational Operator3/2, Product1/3
  Product2/1 -> Add3/3
  Product/1 -> Add3/1
  x_reset/1 -> Product2/1
  Zero-Order Hold/1 -> Add2/1, Add1/2

== system Microgrid_transition_model_092221/Wind Turbine Type 4/Control/Grid-Side Inverter Control/PI with anti-windup and dynamic limits - Iq ==
  note: Aramis Schwanka Trevisan - 16.08.2016
      | PI-controller with anti-windup and dynamic limits
      | Update 17.12.2016: External reset
      | Update 21.02.2017: External reset + limitation
  UpperLimit : Inport
  Input : Inport  Port=2
  LowerLimit : Inport  Port=3
  Reset : Inport  Port=4
  x_reset : Inport  Port=5
  Add1 : Sum
  Add2 : Sum
  Add3 : Sum  Inputs=+++
  Compare To Zero : simulink/Logic and Bit Operations/Compare To Zero  relop=>  OutDataTypeStr=uint8  ZeroCross=off
  Compare To Zero1 : simulink/Logic and Bit Operations/Compare To Zero  relop=<  OutDataTypeStr=uint8  ZeroCross=off
  Constant : Constant  Value=0
  Discrete Integrator : DiscreteIntegrator  IntegratorMethod=Integration: Trapezoidal  gainval=1  ExternalReset=sampled level  InitialConditionSource=external  InitialCondition=Init  SampleTime=Ts  UpperSaturationLimit=UpperLimit  LowerSaturationLimit=LowerLimit  ShowStatePort=on  ICPrevOutput=DiscIntNeverNeededParam  ICPrevScaledInput=DiscIntNeverNeededParam
  IC : InitialCondition  Value=Init
  Kp1 : Gain  Gain=Kp  SaturateOnIntegerOverflow=on  SampleTime=Ts  OutDataTypeStr=Inherit: Same as input  ParamDataTypeStr=Inherit: Same as input
  Kp5 : Gain  Gain=Ki  SaturateOnIntegerOverflow=on  SampleTime=Ts  OutDataTypeStr=Inherit: Same as input  ParamDataTypeStr=Inherit: Same as input
  Logical Operator : Logic  AllPortsSameDT=off  OutDataTypeStr=boolean
  Logical Operator1 : Logic  AllPortsSameDT=off  OutDataTypeStr=boolean
  Logical Operator2 : Logic  Operator=OR  AllPortsSameDT=off  OutDataTypeStr=boolean
  Logical Operator3 : Logic  Operator=OR  Inputs=3  AllPortsSameDT=off  OutDataTypeStr=boolean
  Logical Operator4 : Logic  Operator=NOT  Inputs=3  AllPortsSameDT=off  OutDataTypeStr=boolean
  Product : Product  Inputs=3
  Product1 : Product  Inputs=3
  Product2 : Product
  Relational Operator : RelationalOperator  OutDataTypeStr=boolean  RndMeth=Nearest
  Relational Operator1 : RelationalOperator  Operator=<=  OutDataTypeStr=boolean  RndMeth=Nearest
  Relational Operator2 : RelationalOperator  OutDataTypeStr=boolean  RndMeth=Nearest
  Relational Operator3 : RelationalOperator  Operator=<=  OutDataTypeStr=boolean  RndMeth=Nearest
  Saturation Dynamic : simulink/Discontinuities/Saturation Dynamic  OutMin=[]  OutMax=[]  OutDataTypeStr=Inherit: Same as second input  OutDataType=fixdt(1, 16)  OutScaling=2^-10  DoSatur=off
  Switch : Switch  Criteria=u2 > Threshold
  Zero-Order Hold : ZeroOrderHold  SampleTime=Ts
  Output : Outport
  wires:
  Saturation Dynamic/1 -> Output/1
  Reset/1 -> Product2/2, Logical Operator3/3, Logical Operator4/1
  IC/1 -> Discrete Integrator/3
  Switch/1 -> Discrete Integrator/1
  Compare To Zero1/1 -> Logical Operator1/2  "Error_is_negative"
  Logical Operator/1 -> Logical Operator2/1
  Relational Operator/1 -> Logical Operator/1  "UpperLimit_is_Reached"
  Relational Operator1/1 -> Logical Operator1/1  "LowerLimit_Is_Reached"
  Logical Operator2/1 -> Switch/2
  Kp1/1 -> Zero-Order Hold/1
  Constant/1 -> Switch/1
  Kp5/1 -> Switch/3
  Add2/1 -> Saturation Dynamic/2
  Zero-Order Hold/1 -> Add2/1, Add1/2
  Add1/1 -> Relational Operator/1, Relational Operator1/1
  Input/1 -> Kp5/1, Compare To Zero1/1, Compare To Zero/1, Kp1/1
  Compare To Zero/1 -> Logical Operator/2  "Error_is_positive"
  Logical Operator1/1 -> Logical Operator2/2
  Relational Operator2/1 -> Logical Operator3/1, Product/2
  Relational Operator3/1 -> Product1/2, Logical Operator3/2
  Logical Operator3/1 -> Discrete Integrator/2
  Add3/1 -> IC/1
  Product1/1 -> Add3/2
  UpperLimit/1 -> Saturation Dynamic/1, Relational Operator/2, Product/1, Relational Operator2/2
  Discrete Integrator/State -> Add1/1, Relational Operator3/1, Relational Operator2/1
  Discrete Integrator/1 -> Add2/2
  Logical Operator4/1 -> Product/3, Product1/1
  LowerLimit/1 -> Saturation Dynamic/3, Relational Operator1/2, Relational Operator3/2, Product1/3
  Product2/1 -> Add3/3
  Product/1 -> Add3/1
  x_reset/1 -> Product2/1

== system Microgrid_transition_model_092221/Wind Turbine Type 4/Control/Grid-Side Inverter Control/Predictor1 ==
  in : Inport
  Delay : Delay  DelayLength=1  InitialCondition=Init_value  SampleTime=Ts
  Delay1 : Delay  DelayLength=1  InitialCondition=Init_value  SampleTime=Ts
  Gain : Gain  Gain=2
  Sum1 : Sum  Inputs=|+-
  out : Outport
  wires:
  in/1 -> Delay/1
  Delay1/1 -> Sum1/2
  Sum1/1 -> out/1
  Delay/1 -> Gain/1, Delay1/1
  Gain/1 -> Sum1/1

== system Microgrid_transition_model_092221/Wind Turbine Type 4/Control/Grid-Side Inverter Control/Predictor2 ==
  in : Inport
  Delay : Delay  DelayLength=1  InitialCondition=Init_value  SampleTime=Ts
  Delay1 : Delay  DelayLength=1  InitialCondition=Init_value  SampleTime=Ts
  Gain : Gain  Gain=2
  Sum1 : Sum  Inputs=|+-
  out : Outport
  wires:
  Gain/1 -> Sum1/1
  Delay/1 -> Delay1/1, Gain/1
  Sum1/1 -> out/1
  Delay1/1 -> Sum1/2
  in/1 -> Delay/1

== system Microgrid_transition_model_092221/Wind Turbine Type 4/Control/Measurement and Transformation/Discrete 3-phase PLL-Driven Positive-Sequence Active & Reactive Power ==
  note: Pierre Giroux, Gilbert Sybille
      | Power System Simulation Laboratory
      | IREQ, Hydro-Quebc
  note: Discrete 3-phase PLL-driven Positive-Sequence Active & Reactive Power
  Freq : Inport  PortDimensions=1
  w : Inport  Port=2  PortDimensions=1
  Vabc : Inport  Port=3  PortDimensions=3
  Iabc : Inport  Port=4  PortDimensions=3
  Deg->Rad : Gain  Gain=pi/180  SaturateOnIntegerOverflow=on  OutDataTypeStr=Inherit: Same as input  ParamDataTypeStr=Inherit: Same as input
  Discrete 3-phase PLL-Driven Positive-Sequence Fundamental Value : Subsystem  mask(Discrete 3-phase PLL-Driven Positive-Sequence Fundamental Value){Finit=Finit, Fmin=Fmin, Par_Init=Par_Vinit, Ts=Ts}
      mask prompts: Finit "Initial frequency (Hz):"; Fmin "Minimum frequency (Hz):"; Par_Init "Initial input (positive component): [ Mag  Phase-relative-to-PLL(degrees) ]"; Ts "Sample time:"
      mask help:
      | For a supplied fundamental frequency (port Freq), this discrete block computes  the positive-sequence component (Magnitude and Phase)  of a set of three balanced or unbalanced signals (port abc) which may contain harmonics.
      |  Input port "Sin_Cos" (a two-dimension signal) provides the reference frame required for the computation..
      |  First and second outputs return respectively the magnitude and phase (in degrees relative to the PLL phase)) of the fundamental.
      | For the first cycle of simulation, the outputs are held constant to the values specified by the parameter "Initial input".
      | constant to the values specified by the parameter "Initial input". The value of the parameter "Minimum frequency" is used to determine the buffer size of the "Variable Transport Delay" block found inside this subsystem.
      mask init:
      | Real_Init=Par_Init(1)*cos(pi/180*Par_Init(2));
      | Imag_Init=Par_Init(1)*sin(pi/180*Par_Init(2));
      | power_initmask();
      settings: OpenFcn=power_openblockproxy();
  Discrete 3-phase PLL-Driven Positive-Sequence Fundamental Value2 : Subsystem  mask(Discrete 3-phase PLL-Driven Positive-Sequence Fundamental Value){Finit=Finit, Fmin=Fmin, Par_Init=Par_Iinit, Ts=Ts}
      mask prompts: Finit "Initial frequency (Hz):"; Fmin "Minimum frequency (Hz):"; Par_Init "Initial input (positive component): [ Mag  Phase-relative-to-PLL(degrees) ]"; Ts "Sample time:"
      mask help:
      | For a supplied fundamental frequency (port Freq), this discrete block computes  the positive-sequence component (Magnitude and Phase)  of a set of three balanced or unbalanced signals (port abc) which may contain harmonics.
      |  Input port "Sin_Cos" (a two-dimension signal) provides the reference frame required for the computation..
      |  First and second outputs return respectively the magnitude and phase (in degrees relative to the PLL phase)) of the fundamental.
      | For the first cycle of simulation, the outputs are held constant to the values specified by the parameter "Initial input".
      | constant to the values specified by the parameter "Initial input". The value of the parameter "Minimum frequency" is used to determine the buffer size of the "Variable Transport Delay" block found inside this subsystem.
      mask init:
      | Real_Init=Par_Init(1)*cos(pi/180*Par_Init(2));
      | Imag_Init=Par_Init(1)*sin(pi/180*Par_Init(2));
      | power_initmask();
      settings: OpenFcn=power_openblockproxy();
  Gain1 : Gain  Gain=3/2  SaturateOnIntegerOverflow=on  OutDataTypeStr=Inherit: Same as input  ParamDataTypeStr=Inherit: Same as input
  Mux2 : Mux  Inputs=2
  Mux3 : Mux  Inputs=2
  Product : Product  InputSameDT=on  SaturateOnIntegerOverflow=on  OutDataTypeStr=Inherit: Same as first input
  Product1 : Product  InputSameDT=on  SaturateOnIntegerOverflow=on  OutDataTypeStr=Inherit: Same as first input
  Product2 : Product  InputSameDT=on  SaturateOnIntegerOverflow=on  OutDataTypeStr=Inherit: Same as first input
  Sum : Sum  Inputs=+-  InputSameDT=on  SaturateOnIntegerOverflow=on  OutDataTypeStr=Inherit: Same as first input
  Trigonometric Function : Trigonometry
  Trigonometric Function1 : Trigonometry  Operator=cos
  Mag_V_I : Outport  VectorParamsAs1DForOutWhenUnconnected=off
  P_Q : Outport  Port=2  VectorParamsAs1DForOutWhenUnconnected=off
  wires:
  Iabc/1 -> Discrete 3-phase PLL-Driven Positive-Sequence Fundamental Value2/3(abc)
  Discrete 3-phase PLL-Driven Positive-Sequence Fundamental Value2/1(Mag) -> Product2/2, Mux3/2
  Product2/1 -> Product1/2, Product/1
  Gain1/1 -> P_Q/1
  Mux3/1 -> Mag_V_I/1
  Product1/1 -> Mux2/2
  Product/1 -> Mux2/1
  Mux2/1 -> Gain1/1
  Trigonometric Function/1 -> Product1/1
  Trigonometric Function1/1 -> Product/2
  Deg->Rad/1 -> Trigonometric Function/1, Trigonometric Function1/1
  Sum/1 -> Deg->Rad/1
  Discrete 3-phase PLL-Driven Positive-Sequence Fundamental Value2/2(Phase) -> Sum/2
  Discrete 3-phase PLL-Driven Positive-Sequence Fundamental Value/1(Mag) -> Product2/1, Mux3/1
  Discrete 3-phase PLL-Driven Positive-Sequence Fundamental Value/2(Phase) -> Sum/1
  w/1 -> Discrete 3-phase PLL-Driven Positive-Sequence Fundamental Value2/2(w), Discrete 3-phase PLL-Driven Positive-Sequence Fundamental Value/2(w)
  Freq/1 -> Discrete 3-phase PLL-Driven Positive-Sequence Fundamental Value2/1(Freq), Discrete 3-phase PLL-Driven Positive-Sequence Fundamental Value/1(Freq)
  Vabc/1 -> Discrete 3-phase PLL-Driven Positive-Sequence Fundamental Value/3(abc)

== system Microgrid_transition_model_092221/Wind Turbine Type 4/Control/Measurement and Transformation/Extract References ==
  v_abc : Inport
  Extract References : Subsystem
  Mux : Mux  Inputs=3
  Voltage and Frequency Protection : Subsystem
  rad/s to Hz : Gain  Gain=1/2/pi
  u_frt_pu : Outport
  protection_u_f : Outport  Port=2
  references : Outport  Port=3
  wires:
  Extract References/4(u_frt_pu) -> u_frt_pu/1
  Extract References/2(wt_ref) -> Mux/2
  Extract References/3(w_ref) -> rad/s to Hz/1, Mux/3
  Mux/1 -> references/1
  [Vpos] -> Voltage and Frequency Protection/1(Vpos)
  [fgrid] -> Voltage and Frequency Protection/2(fgrid)
  Voltage and Frequency Protection/1(u_f_protect) -> protection_u_f/1
  Extract References/1(u_ref) -> [Vpos], Mux/1
  rad/s to Hz/1 -> [fgrid]
  v_abc/1 -> Extract References/1(v_abc)

== system Microgrid_transition_model_092221/Wind Turbine Type 4/Control/Measurement and Transformation/Filter ==
  Vabc_grid : Inport
  Iabc_grid_conv : Inport  Port=2
  Vabc_LL_s : Inport  Port=3
  Iabc_stator : Inport  Port=4
  IL : Inport  Port=5
  Vdc : Inport  Port=6
  Qref : Inport  Port=7
  wr : Inport  Port=8
  angle_rotor : Inport  Port=9
  Second-Order Filter{,1..6} (7 alike) : powerlib_meascontrol/Filters/Second-Order Filter  FilterType=Lowpass  Fo=Freq  Zeta=Zeta  Ts=Ts  Initialize=off  Vac_Init="[0,  0,  60]"  Vdc_Init=0  PlotResponse=off  FreqRange=[0, 500, 1]
      settings: SourceProductBaseCode=MT,PS
  Second-Order Filter7 : powerlib_meascontrol/Filters/Second-Order Filter  FilterType=Lowpass  Fo=Freq  Zeta=Zeta  Ts=Ts  Initialize=on  Vac_Init=[0.8 -25 60]*0  Vdc_Init=Vdc_nom  PlotResponse=off  FreqRange=[0, 500, 1]
      settings: SourceProductBaseCode=MT,PS
  Second-Order Filter8 : powerlib_meascontrol/Filters/Second-Order Filter  FilterType=Lowpass  Fo=Freq  Zeta=Zeta  Ts=Ts  Initialize=on  Vac_Init=[0.8 -25 60]*0  Vdc_Init=1+init(1)/100  PlotResponse=off  FreqRange=[0, 500, 1]
      settings: SourceProductBaseCode=MT,PS
  "Vabc_grid " : Outport  VectorParamsAs1DForOutWhenUnconnected=off
  "Iabc_grid_conv " : Outport  Port=2  VectorParamsAs1DForOutWhenUnconnected=off
  "Vabc_LL_s " : Outport  Port=3  VectorParamsAs1DForOutWhenUnconnected=off
  "Iabc_stator " : Outport  Port=4  VectorParamsAs1DForOutWhenUnconnected=off
  "IL " : Outport  Port=5  VectorParamsAs1DForOutWhenUnconnected=off
  "Vdc " : Outport  Port=6  VectorParamsAs1DForOutWhenUnconnected=off
  "Qref " : Outport  Port=7  VectorParamsAs1DForOutWhenUnconnected=off
  "wr " : Outport  Port=8  VectorParamsAs1DForOutWhenUnconnected=off
  "angle_rotor " : Outport  Port=9  VectorParamsAs1DForOutWhenUnconnected=off
  wires:
  angle_rotor/1 -> Second-Order Filter6/1
  Second-Order Filter6/1 -> "angle_rotor "/1
  Second-Order Filter/1 -> "Vabc_grid "/1
  Second-Order Filter1/1 -> "Iabc_grid_conv "/1
  Vdc/1 -> Second-Order Filter7/1
  Second-Order Filter7/1 -> "Vdc "/1
  Second-Order Filter3/1 -> "Iabc_stator "/1
  wr/1 -> Second-Order Filter8/1
  Second-Order Filter8/1 -> "wr "/1
  Qref/1 -> Second-Order Filter5/1
  Second-Order Filter5/1 -> "Qref "/1
  IL/1 -> Second-Order Filter4/1
  Second-Order Filter4/1 -> "IL "/1
  Vabc_grid/1 -> Second-Order Filter/1
  Iabc_grid_conv/1 -> Second-Order Filter1/1
  Vabc_LL_s/1 -> Second-Order Filter2/1
  Second-Order Filter2/1 -> "Vabc_LL_s "/1
  Iabc_stator/1 -> Second-Order Filter3/1
